simulink model "CAN_new"  (R2013b)
settings: Solver=FixedStepDiscrete  StartTime=0.0  StopTime=Inf  FixedStep=0.001  RelTol=1e-3
PostLoadFcn:
  | , if any(exist('dsrtsu_mdlpostloadfcn', 'file') == [2, 3, 6]), try dsrtsu_mdlpostloadfcn('Execute', bdroot); catch fprintf('Error in PostLoadFcn (dsrtsu_mdlpostloadfcn) for model "%s":\n %s\n', bdroot, lasterr); end, end,
undefined symbols (not defined in the file or in its folder): rticanmm_blockfcn, rticanmm_initfcn
libraries: rtimmsu_dsrtlib x4
(part 2 of 2)

== system CAN_new/RTI Data/RTI Data Store ==
  RTI Data Store : Subsystem  mask(RTI_DATA_STORE){}
      mask help:
      | RTI Data Store Block. This block is used by RTI to store internal model dependent data. Deleting this block will result in data loss.
      |
      | NEVER DELETE, COPY, OR MODIFY THIS BLOCK!
      mask Help:
      | RTI Data Store Block. This block is used by RTI to store internal model dependent data. Deleting this block will result in data loss.
      | 
      | NEVER DELETE, COPY, OR MODIFY THIS BLOCK!
      mask Display: text(0.5, 0.5, ' ', 'HorizontalAlignment', 'center');

== system CAN_new/Angle_Sensor/RTICANMM ControllerSetup/ModelClose ==

== system CAN_new/Angle_Sensor/RTICANMM GeneralSetup/ModelClose ==

== system CAN_new/Angle_Sensor/RTICANMM MainBlock/ModelClose ==

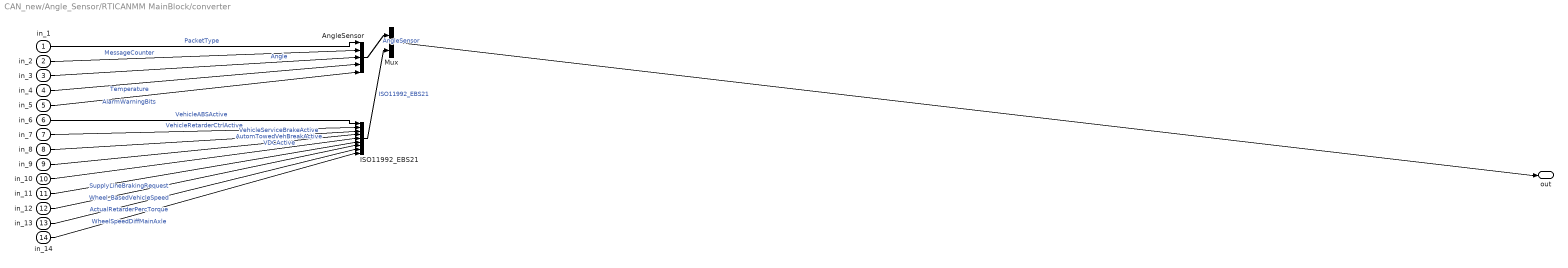
== system CAN_new/Angle_Sensor/RTICANMM MainBlock/converter ==
  in_1 : Inport
  in_2 : Inport  Port=2
  in_3 : Inport  Port=3
  in_4 : Inport  Port=4
  in_5 : Inport  Port=5
  in_6 : Inport  Port=6
  in_7 : Inport  Port=7
  in_8 : Inport  Port=8
  in_9 : Inport  Port=9
  in_10 : Inport  Port=10
  in_11 : Inport  Port=11
  in_12 : Inport  Port=12
  in_13 : Inport  Port=13
  in_14 : Inport  Port=14
  AngleSensor : BusCreator  Inputs=5
  ISO11992_EBS21 : BusCreator  Inputs=9
  Mux : BusCreator  Inputs=2
  out : Outport
  wires:
  in_1/1 -> AngleSensor/1  "PacketType"
  AngleSensor/1 -> Mux/1  "AngleSensor"
  in_2/1 -> AngleSensor/2  "MessageCounter"
  in_3/1 -> AngleSensor/3  "Angle"
  in_4/1 -> AngleSensor/4  "Temperature"
  in_5/1 -> AngleSensor/5  "AlarmWarningBits"
  in_6/1 -> ISO11992_EBS21/1  "VehicleABSActive"
  ISO11992_EBS21/1 -> Mux/2  "ISO11992_EBS21"
  in_7/1 -> ISO11992_EBS21/2  "VehicleRetarderCtrlActive"
  in_8/1 -> ISO11992_EBS21/3  "VehicleServiceBrakeActive"
  in_9/1 -> ISO11992_EBS21/4  "AutomTowedVehBreakActive"
  in_10/1 -> ISO11992_EBS21/5  "VDCActive"
  in_11/1 -> ISO11992_EBS21/6  "SupplyLineBrakingRequest"
  in_12/1 -> ISO11992_EBS21/7  "Wheel_BasedVehicleSpeed"
  in_13/1 -> ISO11992_EBS21/8  "ActualRetarderPercTorque"
  in_14/1 -> ISO11992_EBS21/9  "WheelSpeedDiffMainAxle"
  Mux/1 -> out/1

== system CAN_new/Arduino/RTICANMM ControllerSetup/ModelClose ==

== system CAN_new/Arduino/RTICANMM MainBlock/ModelClose ==

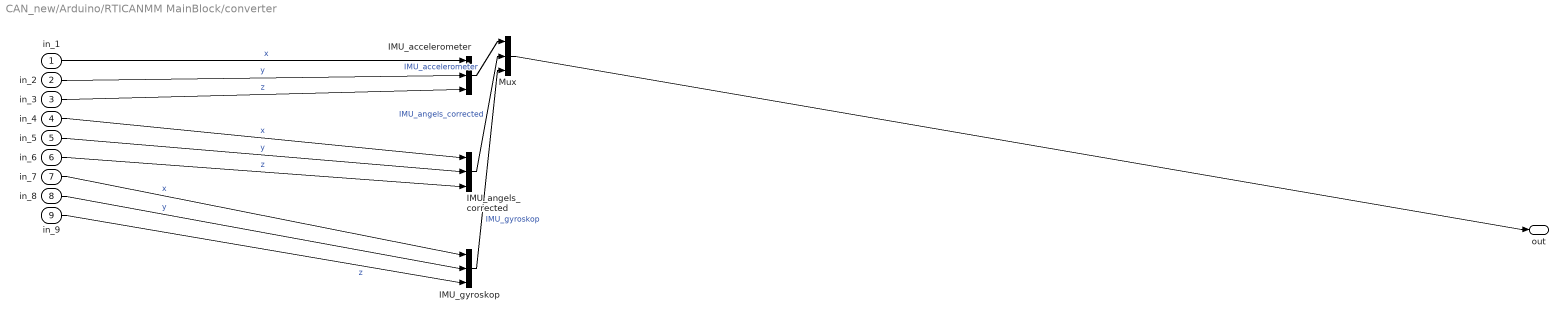
== system CAN_new/Arduino/RTICANMM MainBlock/converter ==
  in_1 : Inport
  in_2 : Inport  Port=2
  in_3 : Inport  Port=3
  in_4 : Inport  Port=4
  in_5 : Inport  Port=5
  in_6 : Inport  Port=6
  in_7 : Inport  Port=7
  in_8 : Inport  Port=8
  in_9 : Inport  Port=9
  IMU_accelerometer : BusCreator  Inputs=3
  IMU_angels_corrected : BusCreator  Inputs=3
  IMU_gyroskop : BusCreator  Inputs=3
  Mux : BusCreator  Inputs=3
  out : Outport
  wires:
  in_1/1 -> IMU_accelerometer/1  "x"
  IMU_accelerometer/1 -> Mux/1  "IMU_accelerometer"
  in_2/1 -> IMU_accelerometer/2  "y"
  in_3/1 -> IMU_accelerometer/3  "z"
  in_4/1 -> IMU_angels_corrected/1  "x"
  IMU_angels_corrected/1 -> Mux/2  "IMU_angels_corrected"
  in_5/1 -> IMU_angels_corrected/2  "y"
  in_6/1 -> IMU_angels_corrected/3  "z"
  in_7/1 -> IMU_gyroskop/1  "x"
  IMU_gyroskop/1 -> Mux/3  "IMU_gyroskop"
  in_8/1 -> IMU_gyroskop/2  "y"
  in_9/1 -> IMU_gyroskop/3  "z"
  Mux/1 -> out/1

== system CAN_new/Arduino/User2RTICANMM MainBlock/IMU_accelerometer ==
  buscreator : BusCreator  Inputs=3
  x : Ground
  y : Ground
  z : Ground
  out : Outport
  wires:
  buscreator/1 -> out/1  "IMU_accelerometer"
  x/1 -> buscreator/1  "x"
  y/1 -> buscreator/2  "y"
  z/1 -> buscreator/3  "z"

== system CAN_new/Arduino/User2RTICANMM MainBlock/IMU_angels_corrected ==
  buscreator : BusCreator  Inputs=3
  x : Ground
  y : Ground
  z : Ground
  out : Outport
  wires:
  buscreator/1 -> out/1  "IMU_angels_corrected"
  x/1 -> buscreator/1  "x"
  y/1 -> buscreator/2  "y"
  z/1 -> buscreator/3  "z"

== system CAN_new/Arduino/User2RTICANMM MainBlock/IMU_gyroskop ==
  buscreator : BusCreator  Inputs=3
  x : Ground
  y : Ground
  z : Ground
  out : Outport
  wires:
  buscreator/1 -> out/1  "IMU_gyroskop"
  x/1 -> buscreator/1  "x"
  y/1 -> buscreator/2  "y"
  z/1 -> buscreator/3  "z"

== system CAN_new/ETS_CAN1/RTICANMM ControllerSetup/ModelClose ==

== system CAN_new/ETS_CAN1/RTICANMM MainBlock/ModelClose ==

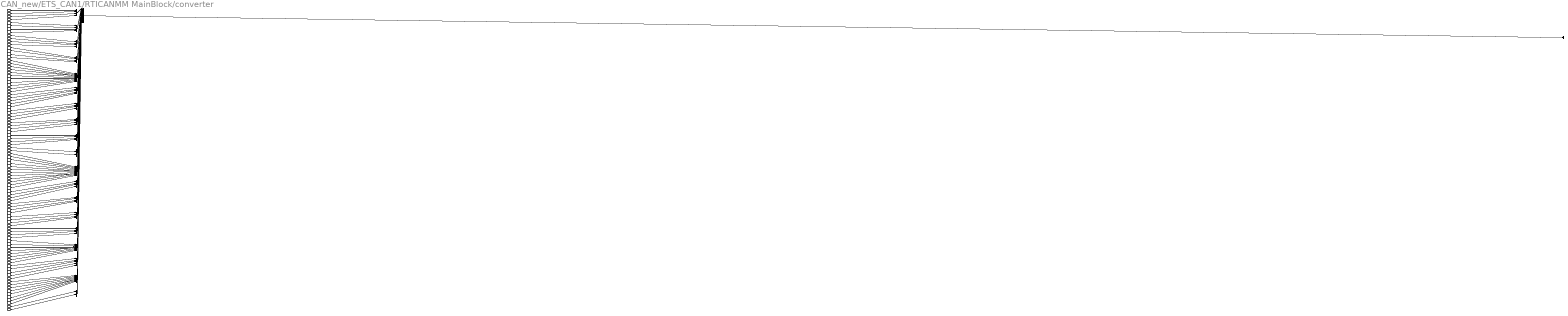
== system CAN_new/ETS_CAN1/RTICANMM MainBlock/converter ==
  in_1 : Inport
  in_2 : Inport  Port=2
  in_3 : Inport  Port=3
  in_4 : Inport  Port=4
  in_5 : Inport  Port=5
  in_6 : Inport  Port=6
  in_7 : Inport  Port=7
  in_8 : Inport  Port=8
  in_9 : Inport  Port=9
  in_10 : Inport  Port=10
  in_11 : Inport  Port=11
  in_12 : Inport  Port=12
  in_13 : Inport  Port=13
  in_14 : Inport  Port=14
  in_15 : Inport  Port=15
  in_16 : Inport  Port=16
  in_17 : Inport  Port=17
  in_18 : Inport  Port=18
  in_19 : Inport  Port=19
  in_20 : Inport  Port=20
  in_21 : Inport  Port=21
  in_22 : Inport  Port=22
  in_23 : Inport  Port=23
  in_24 : Inport  Port=24
  in_25 : Inport  Port=25
  in_26 : Inport  Port=26
  in_27 : Inport  Port=27
  in_28 : Inport  Port=28
  in_29 : Inport  Port=29
  in_30 : Inport  Port=30
  in_31 : Inport  Port=31
  in_32 : Inport  Port=32
  in_33 : Inport  Port=33
  in_34 : Inport  Port=34
  in_35 : Inport  Port=35
  in_36 : Inport  Port=36
  in_37 : Inport  Port=37
  in_38 : Inport  Port=38
  in_39 : Inport  Port=39
  in_40 : Inport  Port=40
  in_41 : Inport  Port=41
  in_42 : Inport  Port=42
  in_43 : Inport  Port=43
  in_44 : Inport  Port=44
  in_45 : Inport  Port=45
  in_46 : Inport  Port=46
  in_47 : Inport  Port=47
  in_48 : Inport  Port=48
  in_49 : Inport  Port=49
  in_50 : Inport  Port=50
  in_51 : Inport  Port=51
  in_52 : Inport  Port=52
  in_53 : Inport  Port=53
  in_54 : Inport  Port=54
  in_55 : Inport  Port=55
  in_56 : Inport  Port=56
  in_57 : Inport  Port=57
  in_58 : Inport  Port=58
  in_59 : Inport  Port=59
  in_60 : Inport  Port=60
  in_61 : Inport  Port=61
  in_62 : Inport  Port=62
  in_63 : Inport  Port=63
  in_64 : Inport  Port=64
  in_65 : Inport  Port=65
  in_66 : Inport  Port=66
  in_67 : Inport  Port=67
  in_68 : Inport  Port=68
  in_69 : Inport  Port=69
  in_70 : Inport  Port=70
  in_71 : Inport  Port=71
  in_72 : Inport  Port=72
  in_73 : Inport  Port=73
  in_74 : Inport  Port=74
  in_75 : Inport  Port=75
  in_76 : Inport  Port=76
  in_77 : Inport  Port=77
  in_78 : Inport  Port=78
  in_79 : Inport  Port=79
  in_80 : Inport  Port=80
  in_81 : Inport  Port=81
  in_82 : Inport  Port=82
  in_83 : Inport  Port=83
  in_84 : Inport  Port=84
  in_85 : Inport  Port=85
  in_86 : Inport  Port=86
  in_87 : Inport  Port=87
  in_88 : Inport  Port=88
  in_89 : Inport  Port=89
  in_90 : Inport  Port=90
  in_91 : Inport  Port=91
  in_92 : Inport  Port=92
  in_93 : Inport  Port=93
  in_94 : Inport  Port=94
  in_95 : Inport  Port=95
  in_96 : Inport  Port=96
  in_97 : Inport  Port=97
  AnalogInputVoltagesMessage1 : BusCreator
  AnalogInputVoltagesMessage2 : BusCreator
  CurrentMeasurementOutputs1 : BusCreator
  CurrentMeasurementOutputs2 : BusCreator
  DigitalInput : BusCreator  Inputs=11
  EtsDataMessage1 : BusCreator  Inputs=5
  EtsDataMessage2 : BusCreator
  EtsDataMessage3 : BusCreator
  EtsDataMessage4 : BusCreator
  EtsDataMessage5 : BusCreator  Inputs=2
  EtsSystemMessage : BusCreator  Inputs=12
  Mux : BusCreator  Inputs=19
  OilSupplyAssignmentMessage : BusCreator
  OilSupplyRequestMessage : BusCreator
  PowersupplyVoltageMessage1 : BusCreator
  PowersupplyVoltageMessage2 : BusCreator
  ResistanceMeasurementOutputs : BusCreator  Inputs=8
  SpeedMessage : BusCreator  Inputs=5
  StatusHighOutputPins : BusCreator  Inputs=8
  StatusLowOutputPins : BusCreator  Inputs=2
  out : Outport
  wires:
  in_1/1 -> AnalogInputVoltagesMessage1/1  "IAV_AIN1_FrontAngle"
  AnalogInputVoltagesMessage1/1 -> Mux/1  "AnalogInputVoltagesMessage1"
  in_2/1 -> AnalogInputVoltagesMessage1/2  "IAV_AIN2_FrontAngleRed"
  in_3/1 -> AnalogInputVoltagesMessage1/3  "IAV_AIN3_RearAngle"
  in_4/1 -> AnalogInputVoltagesMessage1/4  "IAV_AIN4_RearAngleRed"
  in_5/1 -> AnalogInputVoltagesMessage2/1  "IAV_AIN5_PressureSensorX"
  AnalogInputVoltagesMessage2/1 -> Mux/2  "AnalogInputVoltagesMessage2"
  in_6/1 -> AnalogInputVoltagesMessage2/2  "IAV_AIN6_PressureSensorY"
  in_7/1 -> AnalogInputVoltagesMessage2/3  "IAV_AIN7_RearAngle2"
  in_8/1 -> AnalogInputVoltagesMessage2/4  "IAV_AIN8_RearAngle2Red"
  in_9/1 -> CurrentMeasurementOutputs1/1  "CMO_Output1"
  CurrentMeasurementOutputs1/1 -> Mux/3  "CurrentMeasurementOutputs1"
  in_10/1 -> CurrentMeasurementOutputs1/2  "CMO_Output2"
  in_11/1 -> CurrentMeasurementOutputs1/3  "CMO_Output3"
  in_12/1 -> CurrentMeasurementOutputs1/4  "CMO_Output4"
  in_13/1 -> CurrentMeasurementOutputs2/1  "CMO_Output5"
  CurrentMeasurementOutputs2/1 -> Mux/4  "CurrentMeasurementOutputs2"
  in_14/1 -> CurrentMeasurementOutputs2/2  "CMO_Output6"
  in_15/1 -> CurrentMeasurementOutputs2/3  "CMO_Output7"
  in_16/1 -> CurrentMeasurementOutputs2/4  "CMO_Output8"
  in_17/1 -> DigitalInput/1  "DIV_DIN1"
  DigitalInput/1 -> Mux/5  "DigitalInput"
  in_18/1 -> DigitalInput/2  "DIV_DIN2"
  in_19/1 -> DigitalInput/3  "DIV_DIN3"
  in_20/1 -> DigitalInput/4  "DIV_DIN4"
  in_21/1 -> DigitalInput/5  "DIV_DIN5"
  in_22/1 -> DigitalInput/6  "DIV_DIN6"
  in_23/1 -> DigitalInput/7  "DIV_DIN7"
  in_24/1 -> DigitalInput/8  "DIV_DIN8"
  in_25/1 -> DigitalInput/9  "DIV_DIN9"
  in_26/1 -> DigitalInput/10  "DIV_DIN10"
  in_27/1 -> DigitalInput/11  "DIV_DIN11"
  in_28/1 -> EtsDataMessage1/1  "ETSD1_InSpeed1"
  EtsDataMessage1/1 -> Mux/6  "EtsDataMessage1"
  in_29/1 -> EtsDataMessage1/2  "ETSD1_InSpeed2"
  in_30/1 -> EtsDataMessage1/3  "ETSD1_TargetAngle"
  in_31/1 -> EtsDataMessage1/4  "ETSD1_FrontAngle"
  in_32/1 -> EtsDataMessage1/5  "ETSD1_RearAngle"
  in_33/1 -> EtsDataMessage2/1  "ETSD2_Target2Angle"
  EtsDataMessage2/1 -> Mux/7  "EtsDataMessage2"
  in_34/1 -> EtsDataMessage2/2  "ETSD2_Rear2Angle"
  in_35/1 -> EtsDataMessage2/3  "ETSD2_PxPressure"
  in_36/1 -> EtsDataMessage2/4  "ETSD2_PyPressure"
  in_37/1 -> EtsDataMessage3/1  "ETSD3_AmbientTemp"
  EtsDataMessage3/1 -> Mux/8  "EtsDataMessage3"
  in_38/1 -> EtsDataMessage3/2  "ETSD3_OilTemp"
  in_39/1 -> EtsDataMessage3/3  "ETSD3_SecMicroVersion"
  in_40/1 -> EtsDataMessage3/4  "ETSD3_NmiNumber"
  in_41/1 -> EtsDataMessage4/1  "ETSD4_CanSensorAngle"
  EtsDataMessage4/1 -> Mux/9  "EtsDataMessage4"
  in_42/1 -> EtsDataMessage4/2  "ETSD4_CanSensorEtsAngle"
  in_43/1 -> EtsDataMessage4/3  "ETSD4_CanSensorTemp"
  in_44/1 -> EtsDataMessage4/4  "ETSD4_CanSensorAlarm"
  in_45/1 -> EtsDataMessage5/1  "ETSD5_Py2Cofa"
  EtsDataMessage5/1 -> Mux/10  "EtsDataMessage5"
  in_46/1 -> EtsDataMessage5/2  "ETSD5_Py2Pressure"
  in_47/1 -> EtsSystemMessage/1  "ETSS_SteeringState"
  EtsSystemMessage/1 -> Mux/11  "EtsSystemMessage"
  in_48/1 -> EtsSystemMessage/2  "ETSS_AlarmState"
  in_49/1 -> EtsSystemMessage/3  "ETSS_DiagnosticState"
  in_50/1 -> EtsSystemMessage/4  "ETSS_CentringState"
  in_51/1 -> EtsSystemMessage/5  "ETSS_SteerMode"
  in_52/1 -> EtsSystemMessage/6  "ETSS_AlarmPriority"
  in_53/1 -> EtsSystemMessage/7  "ETSS_AlarmReaction"
  in_54/1 -> EtsSystemMessage/8  "ETSS_EtsSimpleStatus"
  in_55/1 -> EtsSystemMessage/9  "ETSS_SupplyVoltageSimpleState"
  in_56/1 -> EtsSystemMessage/10  "ETSS_SpeedSignalSimpleStatus"
  in_57/1 -> EtsSystemMessage/11  "ETSS_KL15State"
  in_58/1 -> EtsSystemMessage/12  "ETSS_TableNumber"
  in_59/1 -> OilSupplyAssignmentMessage/1  "OSAM_Press"
  OilSupplyAssignmentMessage/1 -> Mux/12  "OilSupplyAssignmentMessage"
  in_60/1 -> OilSupplyAssignmentMessage/2  "OSAM_Flow"
  in_61/1 -> OilSupplyAssignmentMessage/3  "OSAM_Pump"
  in_62/1 -> OilSupplyAssignmentMessage/4  "OSAM_Prio"
  in_63/1 -> OilSupplyRequestMessage/1  "OSRM_Press"
  OilSupplyRequestMessage/1 -> Mux/13  "OilSupplyRequestMessage"
  in_64/1 -> OilSupplyRequestMessage/2  "OSRM_Flow"
  in_65/1 -> OilSupplyRequestMessage/3  "OSRM_Pump"
  in_66/1 -> OilSupplyRequestMessage/4  "OSRM_Prio"
  in_67/1 -> PowersupplyVoltageMessage1/1  "PSV_SupV1_KL15"
  PowersupplyVoltageMessage1/1 -> Mux/14  "PowersupplyVoltageMessage1"
  in_68/1 -> PowersupplyVoltageMessage1/2  "PSV_SupV2_KL30"
  in_69/1 -> PowersupplyVoltageMessage1/3  "PSV_SupV3_KL1530"
  in_70/1 -> PowersupplyVoltageMessage1/4  "PSV_SupV4_Internal5V"
  in_71/1 -> PowersupplyVoltageMessage2/1  "PSV_SupV5_Internal6V"
  PowersupplyVoltageMessage2/1 -> Mux/15  "PowersupplyVoltageMessage2"
  in_72/1 -> PowersupplyVoltageMessage2/2  "PSV_SupV6_2VRef"
  in_73/1 -> PowersupplyVoltageMessage2/3  "PSV_SupV7_AngleSensor"
  in_74/1 -> PowersupplyVoltageMessage2/4  "PSV_SupV8_PressureSensor"
  in_75/1 -> ResistanceMeasurementOutputs/1  "RMO_Output1"
  ResistanceMeasurementOutputs/1 -> Mux/16  "ResistanceMeasurementOutputs"
  in_76/1 -> ResistanceMeasurementOutputs/2  "RMO_Output2"
  in_77/1 -> ResistanceMeasurementOutputs/3  "RMO_Output3"
  in_78/1 -> ResistanceMeasurementOutputs/4  "RMO_Output4"
  in_79/1 -> ResistanceMeasurementOutputs/5  "RMO_Output5"
  in_80/1 -> ResistanceMeasurementOutputs/6  "RMO_Output6"
  in_81/1 -> ResistanceMeasurementOutputs/7  "RMO_Output7"
  in_82/1 -> ResistanceMeasurementOutputs/8  "RMO_Output8"
  in_83/1 -> SpeedMessage/1  "SPEED_EtsSpeed"
  SpeedMessage/1 -> Mux/17  "SpeedMessage"
  in_84/1 -> SpeedMessage/2  "SPEED_SecondMicroSpeed"
  in_85/1 -> SpeedMessage/3  "SPEED_MidPointHysteresis"
  in_86/1 -> SpeedMessage/4  "SPEED_SpeedValidIndication"
  in_87/1 -> SpeedMessage/5  "SPEED_LeadSpeed"
  in_88/1 -> StatusHighOutputPins/1  "SHO_Output1"
  StatusHighOutputPins/1 -> Mux/18  "StatusHighOutputPins"
  in_89/1 -> StatusHighOutputPins/2  "SHO_Output2"
  in_90/1 -> StatusHighOutputPins/3  "SHO_Output3"
  in_91/1 -> StatusHighOutputPins/4  "SHO_Output4"
  in_92/1 -> StatusHighOutputPins/5  "SHO_Output5"
  in_93/1 -> StatusHighOutputPins/6  "SHO_Output6"
  in_94/1 -> StatusHighOutputPins/7  "SHO_Output7"
  in_95/1 -> StatusHighOutputPins/8  "SHO_Output8"
  in_96/1 -> StatusLowOutputPins/1  "SLO_Output1"
  StatusLowOutputPins/1 -> Mux/19  "StatusLowOutputPins"
  in_97/1 -> StatusLowOutputPins/2  "SLO_Output2"
  Mux/1 -> out/1

== system CAN_new/RTI Data/RTI Data Store/RTI Data Store ==
  RTI Data Store : Subsystem  mask(RTI_DATA_STORE){}
      mask help:
      | RTI Data Store Block. This block is used by RTI to store internal model dependent data. Deleting this block will result in data loss.
      |
      | NEVER DELETE, COPY, OR MODIFY THIS BLOCK!
      mask Help:
      | RTI Data Store Block. This block is used by RTI to store internal model dependent data. Deleting this block will result in data loss.
      | 
      | NEVER DELETE, COPY, OR MODIFY THIS BLOCK!
      mask Display: text(0.5, 0.5, ' ', 'HorizontalAlignment', 'center');

== system CAN_new/RTI Data/RTI Data Store/RTI Data Store/RTI Data Store ==
  RTI Data Store : Subsystem  mask(RTI_DATA_STORE){}
      mask help:
      | RTI Data Store Block. This block is used by RTI to store internal model dependent data. Deleting this block will result in data loss.
      |
      | NEVER DELETE, COPY, OR MODIFY THIS BLOCK!
      mask Help:
      | RTI Data Store Block. This block is used by RTI to store internal model dependent data. Deleting this block will result in data loss.
      | 
      | NEVER DELETE, COPY, OR MODIFY THIS BLOCK!
      mask Display: text(0.5, 0.5, ' ', 'HorizontalAlignment', 'center');

== system CAN_new/RTI Data/RTI Data Store/RTI Data Store/RTI Data Store/RTI Data Store ==
